simulink library "Lib_Vol_VolumeVar_TMATS"  (R2015a)
settings: Solver=ode45  StartTime=0.0  StopTime=10.0  RelTol=1e-3
undefined symbols (not defined in the file): Fluid
libraries: Lib_Vol_PropLookup_TMATS x1
Description:
  | Thomas Modules
settings Model: CovSFcnEnable=off  Creator=jwchapm2  LastModifiedBy=jwchapm2
settings OptimizationCC: ExpressionDepthLimit=2147483647
settings DebuggingCC: UnderspecifiedInitializationDetection=Classic  MergeDetectMultiDrivingBlocksExec=none  SolverPrmCheckMsg=warning  StateNameClashWarn=warning

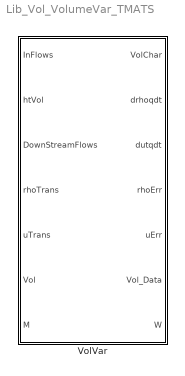
== system Lib_Vol_VolumeVar_TMATS ==
  VolVar : Subsystem  mask(T-MATS: Volume_var Library Block){volume_M=21.3, MolarMass_M=170.33484, htVec_M=Fluid.Vec.ht, PtVec_M=Fluid.Vec.Pt, TtArray_M=Fluid.Array.Tt, uArray_M=Fluid.Array.u, rhoArray_M=Fluid.Array.rho}
      mask prompts: volume_M "volume_M - Volume"; MolarMass_M "MolarMass_M - molar mass"; htVec_M "htVec_M - enthalpy Vector"; PtVec_M "PtVec_M - Pressure Vector"; TtArray_M "TtArray_M - Total Temparture Array f(ht,Pt)"; uArray_M "uArray_M - interal energy Array f(ht,Pt)"; rhoArray_M "rhoArray_M - density Array f(ht,Pt)"
      mask help: This block simulates the performance of a variable volume component using basic fluid dynamic equations and properties.
      mask Help: web(which('Vol_TMATS_VolVar.html'),'-helpbrowser')

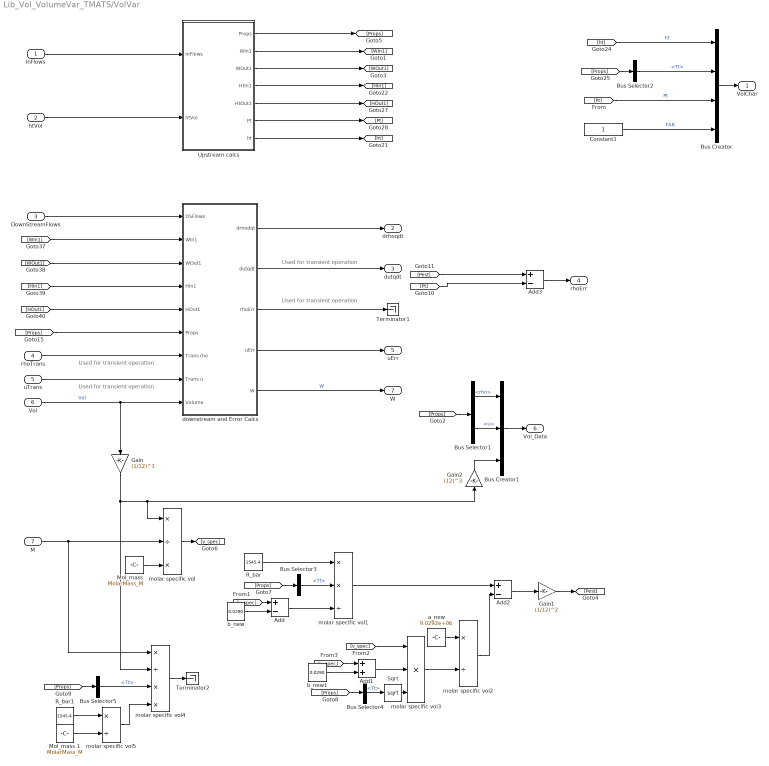
== system Lib_Vol_VolumeVar_TMATS/VolVar ==
  note: Used for transient operation
  note: Used for transient operation
  note: Used for transient operation
  note: Used for transient operation
  InFlows : Inport
  htVol : Inport  Port=2
  DownStreamFlows : Inport  Port=3
  rhoTrans : Inport  Port=4
  uTrans : Inport  Port=5
  Vol : Inport  Port=6
  M : Inport  Port=7
  Add : Sum  Inputs=+-
  Add1 : Sum
  Add2 : Sum  Inputs=+-
  Add3 : Sum  Inputs=+-
  Bus Creator : BusCreator
  Bus Creator1 : BusCreator  Inputs=3
  Bus Selector1 : BusSelector  OutputSignals=rho,u
  Bus Selector{2..5} (4 alike) : BusSelector  OutputSignals=Tt
  Constant1 : Constant
  Gain : Gain  Gain=(1/12)^3
  Gain1 : Gain  Gain=(1/12)^2
  Gain2 : Gain  Gain=(12)^3
  "Mol_mass " : Constant  Value=MolarMass_M
  Mol_mass 1 : Constant  Value=MolarMass_M
  R_bar : Constant  Value=1545.4
  R_bar1 : Constant  Value=1545.4
  Sqrt : Sqrt  SaturateOnIntegerOverflow=on
  Terminator1 : Terminator
  Terminator2 : Terminator
  Upstream calcs : Subsystem  TreatAsAtomicUnit=on
  a_new : Constant  Value=9.0292e+06
  b_new : Constant  Value=0.0290
  b_new1 : Constant  Value=0.0290
  downstream and Error Calcs : Subsystem  TreatAsAtomicUnit=on
  molar specific vol : Product  Inputs=*/*
  molar specific vol1 : Product  Inputs=**/
  molar specific vol2 : Product  Inputs=*/
  molar specific vol3 : Product  Inputs=***
  molar specific vol4 : Product  Inputs=*/**
  molar specific vol5 : Product  Inputs=*/
  VolChar : Outport  PortDimensions=4
  drhoqdt : Outport  Port=2  PortDimensions=1
  dutqdt : Outport  Port=3  PortDimensions=1
  rhoErr : Outport  Port=4  PortDimensions=1
  uErr : Outport  Port=5  PortDimensions=1
  Vol_Data : Outport  Port=6
  W : Outport  Port=7  PortDimensions=1
  wires:
  [Pest] -> Add3/1
  Add3/1 -> rhoErr/1
  [Pt] -> Add3/2
  [Props] -> downstream and Error Calcs/6(Props)
  Gain2/1 -> Bus Creator1/3
  Gain1/1 -> [Pest]
  molar specific vol5/1 -> molar specific vol4/4
  Mol_mass 1/1 -> molar specific vol5/2
  R_bar1/1 -> molar specific vol5/1
  molar specific vol4/1 -> Terminator2/1
  Bus Selector5/1 -> molar specific vol4/3  "<Tt>"
  [Props] -> Bus Selector5/1
  Gain/1 -> Gain2/1, molar specific vol/1, molar specific vol4/2
  molar specific vol2/1 -> Add2/2
  molar specific vol1/1 -> Add2/1
  Add2/1 -> Gain1/1
  Sqrt/1 -> molar specific vol3/3
  molar specific vol3/1 -> molar specific vol2/2
  Add1/1 -> molar specific vol3/2
  [v_spec] -> molar specific vol3/1
  Bus Selector4/1 -> Sqrt/1  "<Tt>"
  [Props] -> Bus Selector4/1
  [v_spec] -> Add1/1
  b_new1/1 -> Add1/2
  a_new/1 -> molar specific vol2/1
  Add/1 -> molar specific vol1/3
  [v_spec] -> Add/1
  b_new/1 -> Add/2
  Bus Selector3/1 -> molar specific vol1/2  "<Tt>"
  [Props] -> Bus Selector3/1
  R_bar/1 -> molar specific vol1/1
  molar specific vol/1 -> [v_spec]
  "Mol_mass "/1 -> molar specific vol/3
  M/1 -> molar specific vol/2, molar specific vol4/1
  rhoTrans/1 -> downstream and Error Calcs/7(Trans rho)
  [Pt] -> Bus Creator/3  "Pt"
  Vol/1 -> Gain/1, downstream and Error Calcs/9(Volume)  "Vol"
  Bus Creator1/1 -> Vol_Data/1
  Bus Selector1/2 -> Bus Creator1/2  "<u>"
  Bus Selector1/1 -> Bus Creator1/1  "<rho>"
  [Props] -> Bus Selector1/1
  InFlows/1 -> Upstream calcs/1(InFlows)
  downstream and Error Calcs/5(W) -> W/1  "W"
  Constant1/1 -> Bus Creator/4  "FAR"
  Upstream calcs/7(ht) -> [ht]
  Bus Selector2/1 -> Bus Creator/2  "<Tt>"
  [Props] -> Bus Selector2/1
  [ht] -> Bus Creator/1  "ht"
  Bus Creator/1 -> VolChar/1
  downstream and Error Calcs/4(uErr) -> uErr/1
  downstream and Error Calcs/3(rhoErr) -> Terminator1/1
  downstream and Error Calcs/2(dutqdt) -> dutqdt/1
  downstream and Error Calcs/1(drhodqt) -> drhoqdt/1
  uTrans/1 -> downstream and Error Calcs/8(Trans u)
  [HOut1] -> downstream and Error Calcs/5(HOut1)
  [HIn1] -> downstream and Error Calcs/4(HIn1)
  [WOut1] -> downstream and Error Calcs/3(WOut1)
  [WIn1] -> downstream and Error Calcs/2(WIn1)
  DownStreamFlows/1 -> downstream and Error Calcs/1(DSFlows)
  Upstream calcs/6(Pt) -> [Pt]
  Upstream calcs/5(HtOut1) -> [HOut1]
  Upstream calcs/4(HtIn1) -> [HIn1]
  Upstream calcs/3(WOut1) -> [WOut1]
  Upstream calcs/2(WIn1) -> [WIn1]
  Upstream calcs/1(Props) -> [Props]
  htVol/1 -> Upstream calcs/2(htVol)

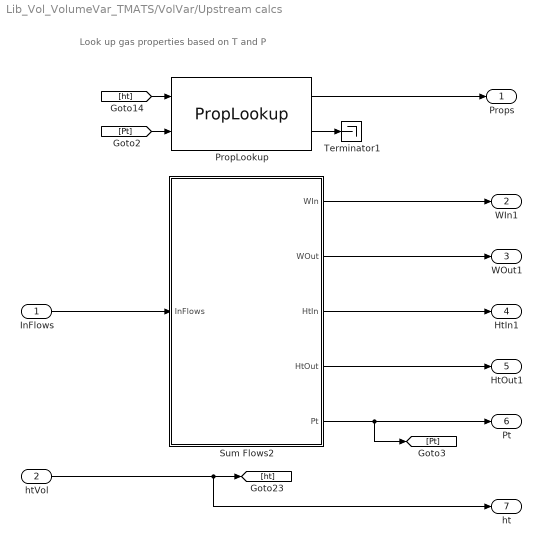
== system Lib_Vol_VolumeVar_TMATS/VolVar/Upstream calcs ==
  note: Look up gas properties based on T and P
  InFlows : Inport
  htVol : Inport  Port=2  PortDimensions=1
  PropLookup : Lib_Vol_PropLookup_TMATS/PropLookup  case_M='ht'  propg_M=0  htg_M=0  htVec_M=htVec_M  PtVec_M=PtVec_M  TtVec_M=[0 10]  sVec_M=[0 10]  htArray_M=ones(2, length(PtVec_M))'  rhoArray_M=rhoArray_M  uArray_M=uArray_M  sArray_M=ones(length(htVec_M), length(PtVec_M))'  muArray_M=ones(length(htVec_M), length(PtVec_M))'  ThArray_M=TtArray_M  CvArray_M=ones(length(htVec_M), length(PtVec_M))'  CpArray_M=ones(length(htVec_M), length(PtVec_M))'  kArray_M=ones(length(htVec_M), length(PtVec_M))'  TsArray_M=ones(2, length(PtVec_M))'  hsArray_M=ones(2, length(PtVec_M))'  Rval_M=Gas.Array.R
  Sum Flows2 : MATLAB Function  TreatAsAtomicUnit=on
  Terminator1 : Terminator
  Props : Outport
  WIn1 : Outport  Port=2
  WOut1 : Outport  Port=3
  HtIn1 : Outport  Port=4
  HtOut1 : Outport  Port=5
  Pt : Outport  Port=6
  ht : Outport  Port=7
  wires:
  Sum Flows2/5(Pt) -> Pt/1, [Pt]
  Sum Flows2/4(HtOut) -> HtOut1/1
  Sum Flows2/3(HtIn) -> HtIn1/1
  Sum Flows2/2(WOut) -> WOut1/1
  Sum Flows2/1(WIn) -> WIn1/1
  InFlows/1 -> Sum Flows2/1(InFlows)
  [ht] -> PropLookup/1
  [Pt] -> PropLookup/2
  PropLookup/2 -> Terminator1/1
  PropLookup/1 -> Props/1
  htVol/1 -> [ht], ht/1

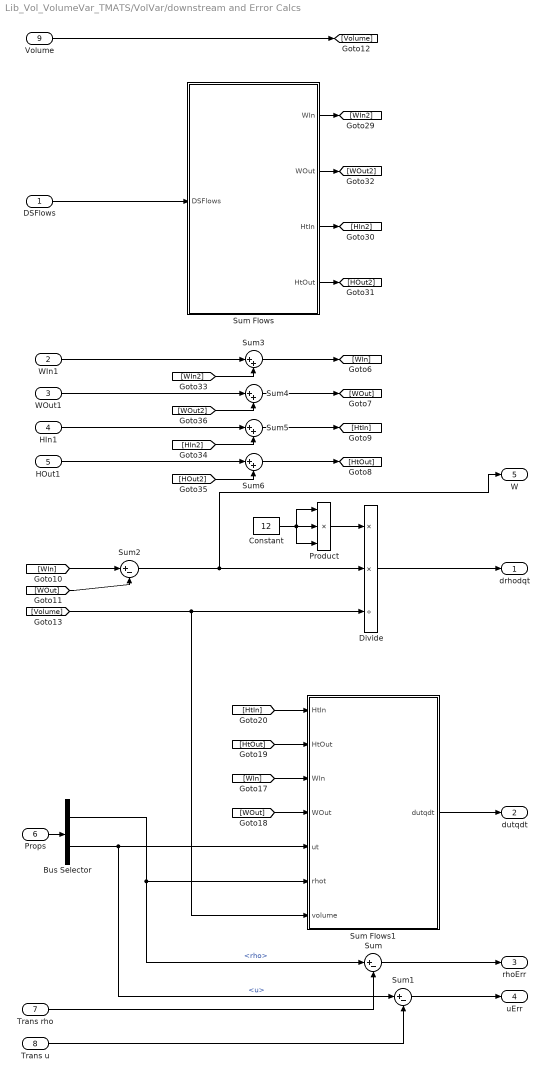
== system Lib_Vol_VolumeVar_TMATS/VolVar/downstream and Error Calcs ==
  DSFlows : Inport
  WIn1 : Inport  Port=2
  WOut1 : Inport  Port=3
  HIn1 : Inport  Port=4
  HOut1 : Inport  Port=5
  Props : Inport  Port=6
  Trans rho : Inport  Port=7
  Trans u : Inport  Port=8
  Volume : Inport  Port=9
  Bus Selector : BusSelector  OutputSignals=rho,u
  Constant : Constant  Value=12
  Divide : Product  Inputs=**/
  Product : Product  Inputs=3
  Sum : Sum  Inputs=|+-
  Sum Flows : MATLAB Function  TreatAsAtomicUnit=on
  Sum Flows1 : MATLAB Function  TreatAsAtomicUnit=on
  Sum1 : Sum  Inputs=|+-
  Sum2 : Sum  Inputs=|+-
  Sum{3..6} (4 alike) : Sum  Inputs=|++
  drhodqt : Outport
  dutqdt : Outport  Port=2
  rhoErr : Outport  Port=3
  uErr : Outport  Port=4
  W : Outport  Port=5
  wires:
  Sum6/1 -> [HtOut]
  Sum5/1 -> [HtIn]
  HIn1/1 -> Sum5/1
  [HIn2] -> Sum5/2
  [HOut2] -> Sum6/2
  HOut1/1 -> Sum6/1
  Sum3/1 -> [WIn]
  Sum4/1 -> [WOut]
  [WOut2] -> Sum4/2
  WOut1/1 -> Sum4/1
  [WIn2] -> Sum3/2
  WIn1/1 -> Sum3/1
  Sum Flows/4(HtOut) -> [HOut2]
  Sum Flows/3(HtIn) -> [HIn2]
  Sum Flows/2(WOut) -> [WOut2]
  Sum Flows/1(WIn) -> [WIn2]
  Sum1/1 -> uErr/1
  Sum/1 -> rhoErr/1
  Sum Flows1/1(dutqdt) -> dutqdt/1
  [HtIn] -> Sum Flows1/1(HtIn)
  [HtOut] -> Sum Flows1/2(HtOut)
  [WOut] -> Sum Flows1/4(WOut)
  [WIn] -> Sum Flows1/3(WIn)
  [Volume] -> Divide/3, Sum Flows1/7(volume)
  Divide/1 -> drhodqt/1
  Volume/1 -> [Volume]
  Product/1 -> Divide/1
  Sum2/1 -> Divide/2, W/1
  Constant/1 -> Product/2, Product/1, Product/3
  [WOut] -> Sum2/2
  [WIn] -> Sum2/1
  Bus Selector/2 -> Sum Flows1/5(ut), Sum1/1  "<u>"
  Bus Selector/1 -> Sum/1, Sum Flows1/6(rhot)  "<rho>"
  Props/1 -> Bus Selector/1
  DSFlows/1 -> Sum Flows/1(DSFlows)
  Trans u/1 -> Sum1/2
  Trans rho/1 -> Sum/2

== matlab function Lib_Vol_VolumeVar_TMATS/VolVar/Upstream calcs/Sum Flows2 ==
  data: WIn output; WOut output; HtIn output; HtOut output; Pt output; InFlows input
function [WIn,WOut, HtIn,HtOut, Pt] = fcn(InFlows)
%#codegen

NumInFlows = length(InFlows)/5;

WIn = 0;
WOut = 0;
HtIn = 0;
HtOut = 0;

for i = 1: NumInFlows
   W = InFlows((i-1)*5 + 1);
   ht = InFlows((i-1)*5 + 2);
   if W > 0 
       WIn = WIn + W;
       HtIn = HtIn + W*ht;
   else 
       WOut = WOut - W;
       HtOut = HtOut - W*ht;
   end
end

Pt = InFlows(4);

== matlab function Lib_Vol_VolumeVar_TMATS/VolVar/downstream and Error Calcs/Sum Flows ==
  data: WIn output; WOut output; HtIn output; HtOut output; DSFlows input
function [WIn,WOut, HtIn,HtOut] = fcn(DSFlows)
%#codegen

NumDSFlows = length(DSFlows)/5;

WIn = 0;
WOut = 0;
HtIn = 0;
HtOut = 0;

for i = 1: NumDSFlows
   W = DSFlows((i-1)*5 + 1);
   ht = DSFlows((i-1)*5 + 2);
   if W > 0 
       WOut = WOut + W;
       HtOut = HtOut + W*ht;
   else 
       WIn = WIn - W;
       HtIn = HtIn - W*ht;
   end
end

== matlab function Lib_Vol_VolumeVar_TMATS/VolVar/downstream and Error Calcs/Sum Flows1 ==
  data: HtIn input; HtOut input; WIn input; WOut input; ut input; dutqdt output; rhot input; volume input
function dutqdt = fcn(HtIn,HtOut, WIn, WOut, ut, rhot, volume)
%#codegen

dutqdt = ( HtIn - HtOut - ut * ( WIn - WOut )) / ( rhot * volume/12/12/12 );
